simulink model "week1_problem9"  (R2020b)
settings: Solver=VariableStepAuto  StartTime=0.0  StopTime=10.0  RelTol=1e-3
libraries: simulink x6
settings Model: Creator=gokul  LastModifiedBy=gokul

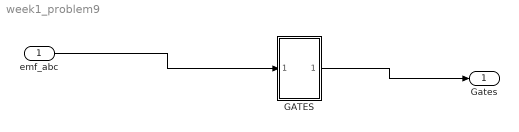
== system week1_problem9 ==
  "emf_abc " : Inport
  GATES : Subsystem
  Gates : Outport
  wires:
  "emf_abc "/1 -> GATES/1(In1)
  GATES/1(Out1) -> Gates/1

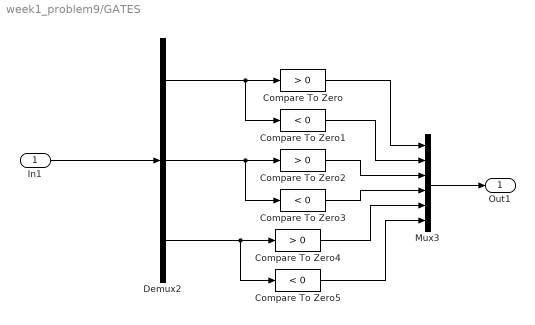
== system week1_problem9/GATES ==
  In1 : Inport
  Compare To Zero : simulink/Logic and Bit Operations/Compare To Zero  relop=>  OutDataTypeStr=boolean  ZeroCross=off
  Compare To Zero1 : simulink/Logic and Bit Operations/Compare To Zero  relop=<  OutDataTypeStr=boolean  ZeroCross=off
  Compare To Zero2 : simulink/Logic and Bit Operations/Compare To Zero  relop=>  OutDataTypeStr=boolean  ZeroCross=off
  Compare To Zero3 : simulink/Logic and Bit Operations/Compare To Zero  relop=<  OutDataTypeStr=boolean  ZeroCross=off
  Compare To Zero4 : simulink/Logic and Bit Operations/Compare To Zero  relop=>  OutDataTypeStr=boolean  ZeroCross=off
  Compare To Zero5 : simulink/Logic and Bit Operations/Compare To Zero  relop=<  OutDataTypeStr=boolean  ZeroCross=off
  Demux2 : Demux  Outputs=3
  Mux3 : Mux  Inputs=6
  Out1 : Outport
  wires:
  Compare To Zero3/1 -> Mux3/4
  Demux2/1 -> Compare To Zero/1, Compare To Zero1/1
  Demux2/3 -> Compare To Zero4/1, Compare To Zero5/1
  Demux2/2 -> Compare To Zero2/1, Compare To Zero3/1
  Compare To Zero5/1 -> Mux3/6
  Compare To Zero2/1 -> Mux3/3
  In1/1 -> Demux2/1
  Compare To Zero1/1 -> Mux3/2
  Compare To Zero4/1 -> Mux3/5
  Compare To Zero/1 -> Mux3/1
  Mux3/1 -> Out1/1
